simulink model "actuator_model"  (R2020b)
settings: Solver=ode4  StartTime=0.0  StopTime=10.0  FixedStep=0.0001  RelTol=1e-3
undefined symbols (not defined in the file): A1, A2, K, m_actuator, V01, V02
settings Model: Creator=HP  LastModifiedBy=HP

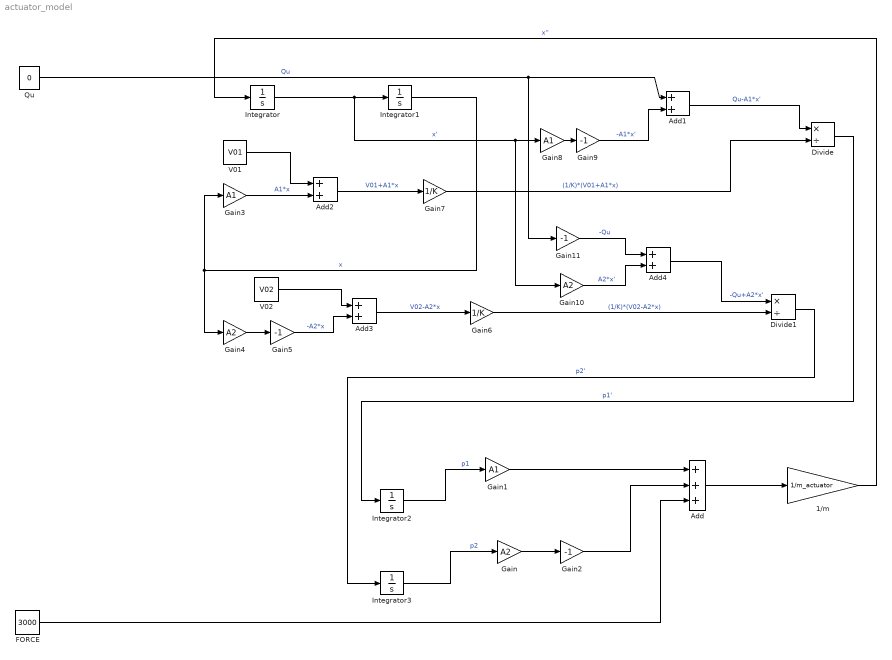
== system actuator_model ==
  1/m : Gain  Gain=1/m_actuator
  Add : Sum  Inputs=+++
  Add{1..4} (4 alike) : Sum
  Divide : Product  Inputs=*/
  Divide1 : Product  Inputs=*/
  FORCE : Constant  Value=3000
  Gain : Gain  Gain=A2
  Gain1 : Gain  Gain=A1
  Gain10 : Gain  Gain=A2
  Gain{2,5,9,11} (4 alike) : Gain  Gain=-1
  Gain3 : Gain  Gain=A1
  Gain4 : Gain  Gain=A2
  Gain6 : Gain  Gain=1/K
  Gain7 : Gain  Gain=1/K
  Gain8 : Gain  Gain=A1
  Integrator{,1..3} (4 alike) : Integrator
  Qu : Constant  Value=0
  V01 : Constant  Value=V01
  V02 : Constant  Value=V02
  wires:
  V02/1 -> Add3/1
  Qu/1 -> Add1/1, Gain11/1  "Qu"
  Integrator1/1 -> Gain3/1, Gain4/1  "x"
  Divide/1 -> Integrator2/1  "p1'"
  FORCE/1 -> Add/3
  Add1/1 -> Divide/1  "Qu-A1*x'"
  Integrator3/1 -> Gain/1  "p2"
  Gain4/1 -> Gain5/1
  Add4/1 -> Divide1/1  "-Qu+A2*x'"
  Add2/1 -> Gain7/1  "V01+A1*x"
  Gain7/1 -> Divide/2  "(1/K)*(V01+A1*x)"
  Integrator2/1 -> Gain1/1  "p1"
  Gain11/1 -> Add4/1  "-Qu"
  Gain10/1 -> Add4/2  "A2*x'"
  Gain8/1 -> Gain9/1
  Gain2/1 -> Add/2
  Divide1/1 -> Integrator3/1  "p2'"
  Gain5/1 -> Add3/2  "-A2*x"
  Gain1/1 -> Add/1
  V01/1 -> Add2/1
  Integrator/1 -> Gain10/1, Gain8/1, Integrator1/1  "x'"
  Gain9/1 -> Add1/2  "-A1*x'"
  Gain/1 -> Gain2/1
  1/m/1 -> Integrator/1  "x''"
  Add/1 -> 1/m/1
  Add3/1 -> Gain6/1  "V02-A2*x"
  Gain6/1 -> Divide1/2  "(1/K)*(V02-A2*x)"
  Gain3/1 -> Add2/2  "A1*x"
